simulink model "IMU_board_example_Sensors_grouped"  (R2017b)
settings: Solver=ode1  StartTime=0.0  StopTime=inf  FixedStep=.004  RelTol=1e-3  EnableMultiTasking=on
undefined symbols (not defined in the file or in its folder): deg, s
libraries: CP_library x1, QB_pacer_lib x1, qbmove_library x1
settings Model: Creator=laurentio  LastModifiedBy=MattiaCP
settings DataIOCC: LimitDataPoints=on  SaveFormat=Array
settings OptimizationCC: LifeSpan=inf
settings DebuggingCC: UnderspecifiedInitializationDetection=Classic  MergeDetectMultiDrivingBlocksExec=none  SolverPrmCheckMsg=warning  AllowSymbolicDim=off  StateNameClashWarn=warning  SFUnexpectedBacktrackingDiag=warning  SFNoUnconditionalDefaultTransitionDiag=warning  SFExecutionAtInitializationDiag=none
settings HardwareCC: ProdBitPerPointer=32  ProdBitPerSizeT=32  ProdBitPerPtrDiffT=32  ProdLargestAtomicFloat=None  ProdIntDivRoundTo=Undefined  ProdEndianess=Unspecified  ProdWordSize=32  ProdHWDeviceType=32-bit Generic
settings ModelReferenceCC: PropagateSignalLabelsOutOfModel=off
settings CodeAppCC: StateflowObjectComments=on
settings GRTTargetCC: TargetLangStandard=C89/C90 (ANSI)  GeneratePreprocessorConditionals=Disable all
settings ConfigComp: CovMetricSettings=dw  CovHtmlReporting=on  CovSaveCumulativeToWorkspaceVar=on  CovSaveSingleToWorkspaceVar=on  CovExternalEMLEnable=off  CovSFcnEnable=off

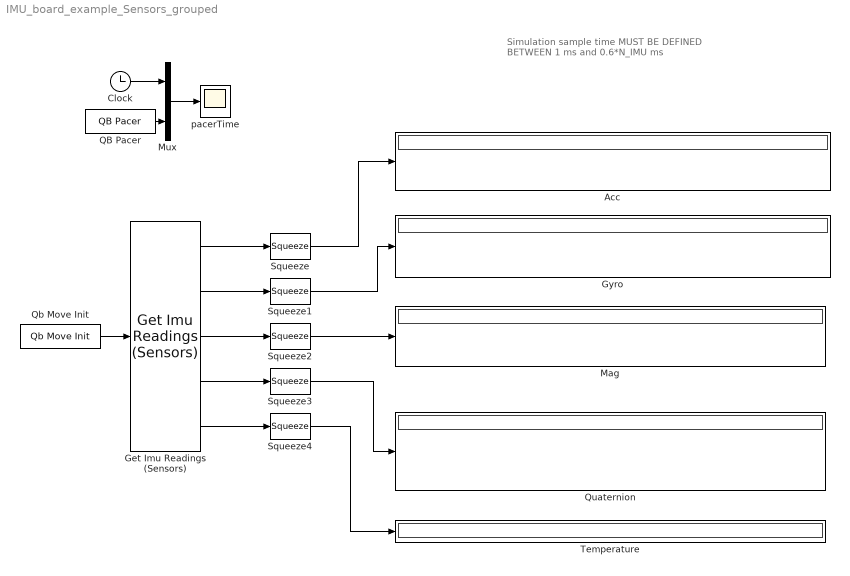
== system IMU_board_example_Sensors_grouped ==
  note: Simulation sample time
      | MUST BE DEFINED BETWEEN
      | 1 ms and 0.6*N_IMU ms
  Acc : Display
  Clock : Clock
  Get Imu Readings (Sensors) : CP_library/Get Imu Readings (Sensors)  ID=1  N_IMU=2  DAISY_CHAINING=off  ACC_UNITY=G  GYRO_UNITY=deg/s  MAG_UNITY=uT
  Gyro : Display
  Mag : Display
  Mux : Mux  Inputs=2
  QB Pacer : QB_pacer_lib/QB Pacer  simTimePerRealTime=1
  Qb Move Init : qbmove_library/Qb Move Init  NUMBER_OF_COM='COM9'  BAUD_RATE_COM=2000000
      settings: SourceProductName=Qb Move Library
  Quaternion : Display
  Squeeze{,1..4} (5 alike) : Squeeze
  Temperature : Display
  pacerTime : Scope
  wires:
  QB Pacer/1 -> Mux/2
  Clock/1 -> Mux/1
  Qb Move Init/1 -> Get Imu Readings (Sensors)/1
  Mux/1 -> pacerTime/1
  Get Imu Readings (Sensors)/1 -> Squeeze/1
  Get Imu Readings (Sensors)/2 -> Squeeze1/1
  Get Imu Readings (Sensors)/3 -> Squeeze2/1
  Get Imu Readings (Sensors)/4 -> Squeeze3/1
  Get Imu Readings (Sensors)/5 -> Squeeze4/1
  Squeeze/1 -> Acc/1
  Squeeze1/1 -> Gyro/1
  Squeeze2/1 -> Mag/1
  Squeeze3/1 -> Quaternion/1
  Squeeze4/1 -> Temperature/1
